simulink model "Cart_Pendulum_n9464263"  (R2020a)
settings: Solver=VariableStepAuto  StartTime=0.0  StopTime=10.0  RelTol=1e-3
undefined symbols (not defined in the file or in its folder): x0
settings Model: Creator=cal  LastModifiedBy=cal
settings DataIOCC: ExternalInput=[m M_c l g]  SaveFormat=Array

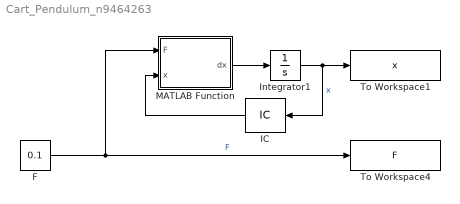
== system Cart_Pendulum_n9464263 ==
  F : Constant  Value=0.1
  IC : InitialCondition  Value=x0
  Integrator1 : Integrator
  MATLAB Function : MATLAB Function  TreatAsAtomicUnit=on
  To Workspace1 : ToWorkspace  VariableName=x  SaveFormat=Timeseries  SampleTime=-1
  To Workspace4 : ToWorkspace  VariableName=F  SaveFormat=Timeseries  SampleTime=-1
  wires:
  F/1 -> MATLAB Function/1(F), To Workspace4/1  "F"
  Integrator1/1 -> IC/1, To Workspace1/1  "x"
  MATLAB Function/1(dx) -> Integrator1/1
  IC/1 -> MATLAB Function/2(x)

== matlab function Cart_Pendulum_n9464263/MATLAB Function ==
  data: F input; dx output; x input
function dx = fcn(F, x)
dx = zeros(size(x));
dx = nonlinear_dynamics(F, x);
